simulink model "Control_Signal_Mapping"  (R2024b)
settings: Solver=VariableStepAuto  StartTime=0.0  StopTime=10.0  RelTol=1e-3  AbsTol=1e-3
model workspace (MAT data in the model file):
  m = 1
undefined symbols (not defined in the file or in its folder): Q_targets, RPM1_grid, RPM2_grid, T_targets
libraries: fl_lib x22, ee_lib x11, nesl_utility x10, sdl_lib x2, slpidlib x2, shared6dof x1, robotcorelib x1, aerolibnav x1, aerolibutil x1, matrix_library x1
(part 2 of 2)

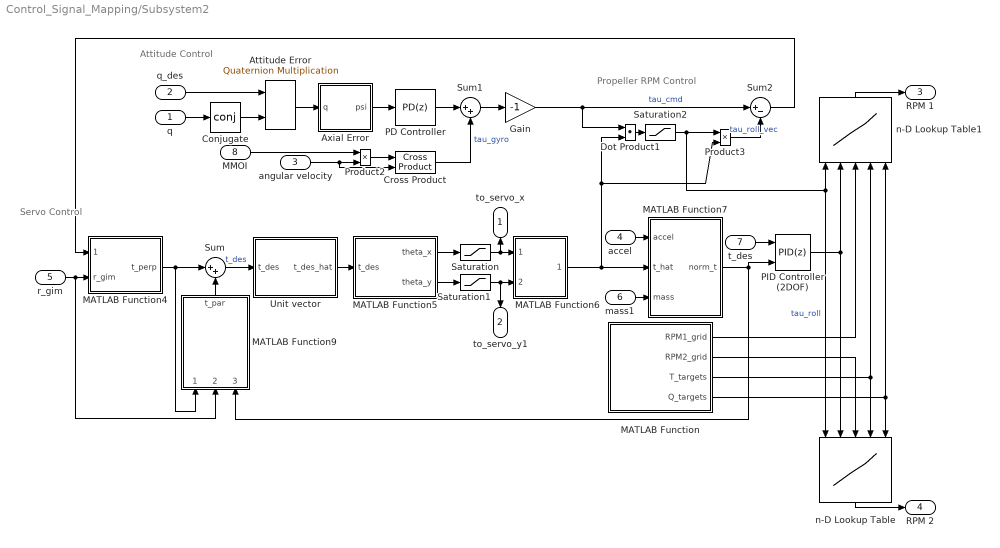
== system Control_Signal_Mapping/Subsystem2 ==
  note: Propeller RPM Control
  note: Attitude Control
  note: Servo Control
  q : Inport  PortDimensions=4
  q_des : Inport  Port=2  PortDimensions=4
  angular velocity : Inport  Port=3  PortDimensions=3
  accel : Inport  Port=4  PortDimensions=3
  r_gim : Inport  Port=5  PortDimensions=3
  mass1 : Inport  Port=6  PortDimensions=1
  t_des : Inport  Port=7  PortDimensions=3
  MMOI : Inport  Port=8
  Attitude Error : aerolibutil/Quaternion Multiplication
  Axial Error : MATLAB Function  TreatAsAtomicUnit=on
  Conjugate : Math  Operator=conj  SignedPower=on  RndMeth=Zero
  Cross Product : matrix_library/Cross Product
  Dot Product1 : DotProduct  OutDataTypeStr=Inherit: Inherit via internal rule
  Gain : Gain  Gain=-1
  MATLAB Function : MATLAB Function  TreatAsAtomicUnit=on
  MATLAB Function4 : MATLAB Function  TreatAsAtomicUnit=on
  MATLAB Function5 : MATLAB Function  TreatAsAtomicUnit=on
  MATLAB Function6 : MATLAB Function  TreatAsAtomicUnit=on
  MATLAB Function7 : MATLAB Function  TreatAsAtomicUnit=on
  MATLAB Function9 : MATLAB Function  TreatAsAtomicUnit=on
  PD Controller : slpidlib/PID Controller  Controller=PD  Form=Parallel  TimeDomain=Discrete-time  UseExternalTs=off  SampleTime=0.001  IntegratorMethod=Forward Euler  FilterMethod=Forward Euler  ControllerParametersSource=internal  P=1  I=1  UseKiTs=off  D=1  UseExternalDerivativeSource=off  N=1  UseFilter=on  TunerSelectOption=Transfer Function Based (PID Tuner App)  InitialConditionSource=internal  InitialConditionForIntegrator=0  InitialConditionForFilter=1  DifferentiatorICPrevScaledInput=0  ExternalReset=none  TrackingMode=off  Kt=1  LimitOutput=on  SatLimitsSource=internal  UpperSaturationLimit=10  LowerSaturationLimit=-10  LinearizeAsGain=off  AntiWindupMode=none  Kb=1  LimitIntegrator=off  UpperIntegratorSaturationLimit=inf  LowerIntegratorSaturationLimit=-inf  POutMin=[]  POutMax=[]  IOutMin=[]  IOutMax=[]  DOutMin=[]  DOutMax=[]  NOutMin=[]  NOutMax=[]  SumOutMin=[]  SumOutMax=[]  SaturationOutMin=[]  SaturationOutMax=[]  PParamMin=[]  PParamMax=[]  IParamMin=[]  IParamMax=[]  DParamMin=[]  DParamMax=[]  NParamMin=[]  NParamMax=[]  KbParamMin=[]  KbParamMax=[]  KtParamMin=[]  KtParamMax=[]  KbOutMin=[]  KbOutMax=[]  KtOutMin=[]  KtOutMax=[]  IntegratorOutMin=[]  IntegratorOutMax=[]  FilterOutMin=[]  FilterOutMax=[]  SumI1OutMin=[]  SumI1OutMax=[]  SumI2OutMin=[]  SumI2OutMax=[]  SumI3OutMin=[]  SumI3OutMax=[]  SumI4OutMin=[]  SumI4OutMax=[]  SumDOutMin=[]  SumDOutMax=[]  DifferentiatorOutMin=[]  DifferentiatorOutMax=[]  FilterDiffOutCoefMin=[]  FilterDiffOutCoefMax=[]  ReciprocalOutMin=[]  ReciprocalOutMax=[]  SumDenOutMin=[]  SumDenOutMax=[]  SumNumOutMin=[]  SumNumOutMax=[]  DivideOutMin=[]  DivideOutMax=[]  UdiffTsProdOutMin=[]  UdiffTsProdOutMax=[]  NTsProdOutMin=[]  NTsProdOutMax=[]  UintegralTsProdOutMin=[]  UintegralTsProdOutMax=[]  UngainTsProdOutMin=[]  UngainTsProdOutMax=[]  ClampingZeroOutDataTypeStr=Inherit: Inherit via back propagation  ClampingZeroOutMin=[]  ClampingZeroOutMax=[]  FilterDenConstantOutDataTypeStr=Inherit: Inherit via back propagation  FilterDenConstantOutMin=[]  FilterDenConstantOutMax=[]  PCopyOutDataTypeStr=Inherit: Inherit via back propagation  PCopyOutMin=[]  PCopyOutMax=[]  NCopyOutDataTypeStr=Inherit: Inherit via back propagation  NCopyOutMin=[]  NCopyOutMax=[]  IntegratorContinuousStateAttributes=''  IntegratorStateMustResolveToSignalObject=off  IntegratorRTWStateStorageClass=Auto  FilterContinuousStateAttributes=''  FilterStateMustResolveToSignalObject=off  FilterRTWStateStorageClass=Auto  ParallelPVariant=InternalParameters  IdealPVariant=Disabled  IVariant=Disabled  DVariant=InternalParameters  IntegratorVariant=Disabled  SatVariant=Enabled  AWVariant=Disabled  PCopyVariant=Disabled  TRVariant=Disabled  FdbkBlocksVariant=Forward  IdealPFdbkVariant=Disabled  SatFdbkVariant=Disabled  DerivativeFilterVariant=ForwardEulerFilter  NVariant=InternalParameters  NCopyVariant=Disabled  FilterICVariant=InternalICsFilter  IntegratorICVariant=Disabled  ExternalResetVariant=Disabled  TRSumVariant=Passthrough  SumFdbkVariant=Disabled  SumVariant=Sum_PD  TsampFilterVariant=InternalTs  TsampNgainVariant=Passthrough  TsampIntegralVariant=Disabled_SignalSpec  ExternalSaturationOutDataTypeStr=Inherit: Same as second input  DerivativeSourceVariant=ErrorSignal  PreIntVariant=InternalPreInt
  PID Controller (2DOF) : slpidlib/PID Controller (2DOF)  Controller=PID  Form=Parallel  TimeDomain=Discrete-time  UseExternalTs=off  SampleTime=-1  IntegratorMethod=Forward Euler  FilterMethod=Forward Euler  ControllerParametersSource=internal  P=1  I=1  UseKiTs=off  D=0  UseExternalDerivativeSource=off  N=100  UseFilter=on  b=1  c=1  TunerSelectOption=Transfer Function Based (PID Tuner App)  InitialConditionSource=internal  InitialConditionForIntegrator=0  InitialConditionForFilter=0  DifferentiatorICPrevScaledInput=0  ExternalReset=none  TrackingMode=off  Kt=1  LimitOutput=off  SatLimitsSource=internal  UpperSaturationLimit=inf  LowerSaturationLimit=-inf  LinearizeAsGain=on  AntiWindupMode=none  Kb=1  LimitIntegrator=off  UpperIntegratorSaturationLimit=inf  LowerIntegratorSaturationLimit=-inf  POutMin=[]  POutMax=[]  IOutMin=[]  IOutMax=[]  DOutMin=[]  DOutMax=[]  NOutMin=[]  NOutMax=[]  bOutMin=[]  bOutMax=[]  cOutMin=[]  cOutMax=[]  SumOutMin=[]  SumOutMax=[]  SaturationOutMin=[]  SaturationOutMax=[]  PParamMin=[]  PParamMax=[]  IParamMin=[]  IParamMax=[]  DParamMin=[]  DParamMax=[]  NParamMin=[]  NParamMax=[]  bParamMin=[]  bParamMax=[]  cParamMin=[]  cParamMax=[]  KbParamMin=[]  KbParamMax=[]  KtParamMin=[]  KtParamMax=[]  KbOutMin=[]  KbOutMax=[]  KtOutMin=[]  KtOutMax=[]  IntegratorOutMin=[]  IntegratorOutMax=[]  FilterOutMin=[]  FilterOutMax=[]  SumI1OutMin=[]  SumI1OutMax=[]  SumI2OutMin=[]  SumI2OutMax=[]  SumI3OutMin=[]  SumI3OutMax=[]  SumI4OutMin=[]  SumI4OutMax=[]  SumDOutMin=[]  SumDOutMax=[]  Sum1OutMin=[]  Sum1OutMax=[]  Sum2OutMin=[]  Sum2OutMax=[]  Sum3OutMin=[]  Sum3OutMax=[]  DifferentiatorOutMin=[]  DifferentiatorOutMax=[]  FilterDiffOutCoefMin=[]  FilterDiffOutCoefMax=[]  ReciprocalOutMin=[]  ReciprocalOutMax=[]  SumDenOutMin=[]  SumDenOutMax=[]  SumNumOutMin=[]  SumNumOutMax=[]  DivideOutMin=[]  DivideOutMax=[]  UdiffTsProdOutMin=[]  UdiffTsProdOutMax=[]  NTsProdOutMin=[]  NTsProdOutMax=[]  UintegralTsProdOutMin=[]  UintegralTsProdOutMax=[]  UngainTsProdOutMin=[]  UngainTsProdOutMax=[]  ClampingZeroOutDataTypeStr=Inherit: Inherit via back propagation  ClampingZeroOutMin=[]  ClampingZeroOutMax=[]  FilterDenConstantOutDataTypeStr=Inherit: Inherit via back propagation  FilterDenConstantOutMin=[]  FilterDenConstantOutMax=[]  PCopyOutDataTypeStr=Inherit: Inherit via back propagation  PCopyOutMin=[]  PCopyOutMax=[]  NCopyOutDataTypeStr=Inherit: Inherit via back propagation  NCopyOutMin=[]  NCopyOutMax=[]  IntegratorContinuousStateAttributes=''  IntegratorStateMustResolveToSignalObject=off  IntegratorRTWStateStorageClass=Auto  FilterContinuousStateAttributes=''  FilterStateMustResolveToSignalObject=off  FilterRTWStateStorageClass=Auto  ParallelPVariant=InternalParameters  IdealPVariant=Disabled  IVariant=InternalParameters  DVariant=InternalParameters  bVariant=InternalParameters  cVariant=InternalParameters  IntegratorVariant=Discrete  SatVariant=Disabled  AWVariant=Passthrough  PCopyVariant=Disabled  TRVariant=Disabled  FdbkBlocksVariant=Forward  IdealPFdbkVariant=Disabled  SatFdbkVariant=Disabled  DerivativeFilterVariant=ForwardEulerFilter  NVariant=InternalParameters  NCopyVariant=Disabled  FilterICVariant=InternalICsFilter  IntegratorICVariant=InternalICs  ExternalResetVariant=Disabled  TRSumVariant=Passthrough  SumFdbkVariant=Disabled  SumVariant=Sum_PID  TsampFilterVariant=InternalTs  TsampNgainVariant=Passthrough  TsampIntegralVariant=Disabled_SignalSpec  ExternalSaturationOutDataTypeStr=Inherit: Same as second input  DerivativeSourceVariant=ErrorSignal  PreIntVariant=InternalPreInt
  Product2 : Product
  Product3 : Product
  Saturation : Saturate
  Saturation1 : Saturate
  Saturation2 : Saturate
  Sum : Sum  Inputs=|++
  Sum1 : Sum  Inputs=|++
  Sum2 : Sum  Inputs=|+-
  Unit vector : MATLAB Function  TreatAsAtomicUnit=on
  n-D Lookup Table : Lookup_n-D  LookupTableObject=''  BreakpointsForDimension1Source=Input port  BreakpointsForDimension1=T_targets  BreakpointsForDimension2Source=Input port  BreakpointsForDimension2=Q_targets  BreakpointsForDimension3=[5, 7]  BreakpointsForDimension1FirstPoint=10  BreakpointsForDimension2FirstPoint=10  BreakpointsForDimension1Spacing=12  BreakpointsForDimension2Spacing=12  TableSource=Input port  Table=RPM2_grid  InternalRulePriority=Speed  RndMeth=Simplest
      settings: InputPortMap=u0,u1,p221,p5,p7
  n-D Lookup Table1 : Lookup_n-D  LookupTableObject=''  BreakpointsForDimension1Source=Input port  BreakpointsForDimension1=T_targets  BreakpointsForDimension2Source=Input port  BreakpointsForDimension2=Q_targets  BreakpointsForDimension3=[5, 7]  BreakpointsForDimension1FirstPoint=10  BreakpointsForDimension2FirstPoint=10  BreakpointsForDimension1Spacing=12  BreakpointsForDimension2Spacing=12  TableSource=Input port  Table=RPM1_grid  InternalRulePriority=Speed  RndMeth=Simplest
      settings: InputPortMap=u0,u1,p221,p5,p7
  to_servo_x : Outport  PortDimensions=1
  to_servo_y1 : Outport  Port=2  PortDimensions=1
  RPM 1 : Outport  Port=3
  RPM 2 : Outport  Port=4
  wires:
  Conjugate/1 -> Attitude Error/2
  MATLAB Function5/1(theta_x) -> Saturation/1
  Attitude Error/1 -> Axial Error/1(q)
  Gain/1 -> Sum2/1, Dot Product1/1  "tau_cmd"
  n-D Lookup Table/1 -> RPM 2/1
  Saturation1/1 -> to_servo_y1/1, MATLAB Function6/2(theta_y)
  Sum/1 -> Unit vector/1(t_des)  "t_des"
  Saturation/1 -> MATLAB Function6/1(theta_x), to_servo_x/1
  Dot Product1/1 -> Saturation2/1
  accel/1 -> MATLAB Function7/1(accel)
  Cross Product/1 -> Sum1/2  "tau_gyro"
  MATLAB Function6/1(t_hat) -> MATLAB Function7/2(t_hat), Dot Product1/2, Product3/2
  MMOI/1 -> Product2/1
  Sum2/1 -> MATLAB Function4/1(tau_gim)
  MATLAB Function4/1(t_perp) -> MATLAB Function9/1(t_perp), Sum/1
  mass1/1 -> MATLAB Function7/3(mass)
  Unit vector/1(t_des_hat) -> MATLAB Function5/1(t_des)
  MATLAB Function5/2(theta_y) -> Saturation1/1
  r_gim/1 -> MATLAB Function9/2(r_gim), MATLAB Function4/2(r_gim)
  q_des/1 -> Attitude Error/1
  Saturation2/1 -> Product3/1, n-D Lookup Table1/1, n-D Lookup Table/1  "tau_roll"
  angular velocity/1 -> Cross Product/2, Product2/2
  Axial Error/1(psi) -> PD Controller/1
  MATLAB Function7/1(norm_t) -> PID Controller (2DOF)/2, MATLAB Function9/3(norm_t)
  Product3/1 -> Sum2/2  "tau_roll_vec"
  Sum1/1 -> Gain/1
  q/1 -> Conjugate/1
  PD Controller/1 -> Sum1/1
  MATLAB Function9/1(t_par) -> Sum/2
  Product2/1 -> Cross Product/1
  n-D Lookup Table1/1 -> RPM 1/1
  t_des/1 -> PID Controller (2DOF)/1
  PID Controller (2DOF)/1 -> n-D Lookup Table/2, n-D Lookup Table1/2
  MATLAB Function/1(RPM1_grid) -> n-D Lookup Table1/3
  MATLAB Function/2(RPM2_grid) -> n-D Lookup Table/3
  MATLAB Function/3(T_targets) -> n-D Lookup Table/4, n-D Lookup Table1/4
  MATLAB Function/4(Q_targets) -> n-D Lookup Table/5, n-D Lookup Table1/5

== matlab function Control_Signal_Mapping/Subsystem/MATLAB Function ==
  data: u input; y output
function y = fcn(u)

y = u;

== matlab function Control_Signal_Mapping/Subsystem2/Unit vector ==
  data: t_des input; t_des_hat output
function t_des_hat = fcn(t_des)
t_des_hat = t_des/norm(t_des);

== matlab function Control_Signal_Mapping/Subsystem2/MATLAB Function4 ==
  data: tau_gim input; t_perp output; r_gim input
function t_perp = fcn(tau_gim, r_gim)

t_perp = (cross(tau_gim, r_gim))/(norm(r_gim)^2);

== matlab function Control_Signal_Mapping/Subsystem2/MATLAB Function5 ==
  data: t_des input; theta_x output; theta_y output
function [theta_x, theta_y] = fcn(t_des)

%theta_x = -atan2(t_des(2), t_des(3)); % t_des(2) and (3) are y and z axes
%theta_y = asin(t_des(1)); % t_des(1) is on x axis 
theta_x = 1;
theta_y = 1;

== matlab function Control_Signal_Mapping/Subsystem2/MATLAB Function6 ==
  data: theta_x input; t_hat output; theta_y input
function t_hat  = fcn(theta_x, theta_y)

t_hat = [sin(theta_y)
    -sin(theta_x)*cos(theta_y)
    cos(theta_x)*cos(theta_y)];

== matlab function Control_Signal_Mapping/Subsystem2/MATLAB Function7 ==
  data: accel input; norm_t output; t_hat input; mass input
function norm_t = fcn(accel, t_hat, mass)

norm_t = mass*(dot(accel, t_hat));

== matlab function Control_Signal_Mapping/Subsystem2/Axial Error ==
  data: q input; psi output
function psi  = fcn(q)

q_0 = q(1);
v = [q(2)
    q(3)
    q(4)];
psi_comp = 2*atan2(norm(v), q_0)*v/norm(v);
psi = sign(psi_comp).*psi_comp;

== matlab function Control_Signal_Mapping/Subsystem2/MATLAB Function9 ==
  data: t_perp input; t_par output; r_gim input; norm_t input
function t_par = fcn(t_perp, r_gim, norm_t)

t_par = sqrt(norm_t^2 - norm(t_perp)^2)*r_gim/norm(r_gim);

== matlab function Control_Signal_Mapping/Subsystem2/MATLAB Function ==
  data: RPM1_grid output; RPM2_grid output; T_targets output; Q_targets output
function [RPM1_grid, RPM2_grid, T_targets, Q_targets] = fcn()

%% Constants for propeller thrust equations (fake, will be replaced by the experimental values)
kT = 1.2e-7;    % Thrust coefficient [N/RPM²]
kQ = 2.0e-9;    % Torque coefficient [N·m/RPM²]
eta = 0.9;      % Efficiency factor for second prop (inflow reduction)

%% RPM ranges (estimated, but can get better with mechanical)
RPM = linspace(0, 30000, 300);
[RPM1, RPM2] = meshgrid(RPM, RPM);

%% Thrust and Torque calculations
T1 = kT .* RPM1.^2;
T2 = kT .* RPM2.^2 .* eta;
T_total = T1 + T2;

Q1 = -kQ .* RPM1.^2;           % CW rotation
Q2 =  kQ .* RPM2.^2 .* eta;    % CCW rotation
Q_total = Q1 + Q2;

%% Flatten grids for fitting
x = RPM1(:);
y = RPM2(:);
z_thrust = T_total(:);
z_torque = Q_total(:);

%% Find the reasonable range for T(thrust) and Q(torque) based on the RPM ranges, whichwe have from mechanical
thrust_max = max(z_thrust);
thrust_min = min(z_thrust);
torque_max = max(z_torque);
torque_min = min(z_torque);

%% 2nd-degree polynomial fitting: z = a + b*x + c*y + d*x^2 + e*x*y + f*y^2
X = [ones(size(x)), x, y, x.^2, x.*y, y.^2];

coeffs_thrust = X \ z_thrust;
coeffs_torque = X \ z_torque;

Z_fit_thrust = reshape(X * coeffs_thrust, size(RPM1));
Z_fit_torque = reshape(X * coeffs_torque, size(RPM1));

%% Target ranges
T_targets = linspace(thrust_min, thrust_max, 100);
Q_targets = linspace(torque_min, torque_max, 100);

%% Initialize result grids
RPM1_grid = nan(length(Q_targets), length(T_targets));
RPM2_grid = nan(length(Q_targets), length(T_targets));


%{
%% Analytical solve
for i = 1:length(Q_targets)
    Q = Q_targets(i);
    for j = 1:length(T_targets)
        T = T_targets(j);
        RPM1_sq = (T/kT - Q/kQ)/2;
        RPM2_sq = (Q + kQ*RPM1_sq) / (kQ * eta);
        if RPM1_sq >= 0 && RPM2_sq >= 0
            RPM1_grid(i,j) = sqrt(RPM1_sq);
            RPM2_grid(i,j) = sqrt(RPM2_sq);
        end
    end
end

%% Replace NaN values with -1 for Simulink compatibility
%%Negative 1 means pair isn't possible
RPM1_grid(isnan(RPM1_grid)) = -1;
RPM2_grid(isnan(RPM2_grid)) = -1;
%}
